simulink model "sampleModel1630_1_sub"  (R2023a)
settings: Solver=VariableStepAuto  StartTime=0.0  StopTime=10.0  RelTol=1e-3
libraries: hdlsllib x3
settings Model: Creator=user1  LastModifiedBy=user1

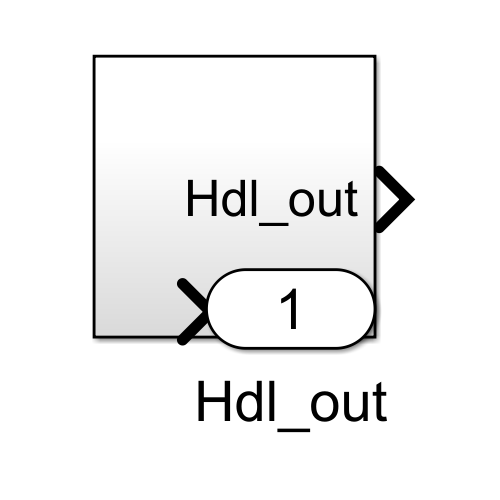
[thumbnail: Simulink's stored preview of the top-level diagram]
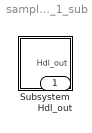
== system sampleModel1630_1_sub ==
  Subsystem : Subsystem
  Hdl_out : Outport  OutDataTypeStr=uint8

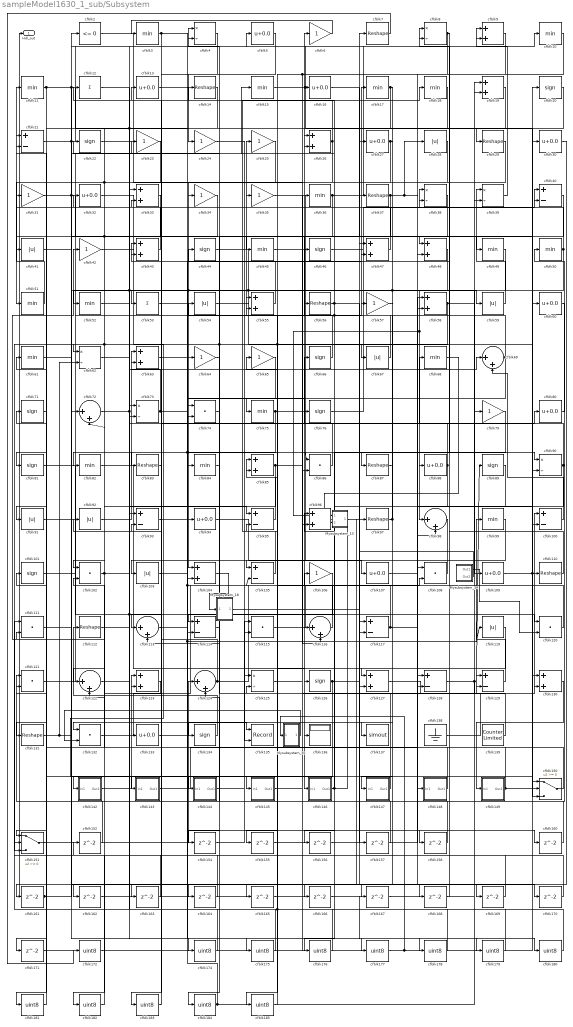
== system sampleModel1630_1_sub/Subsystem ==
  Mysubsystem_13 : Subsystem  TreatAsAtomicUnit=on  RTWFcnName=Mysubsystem_13
      settings: RTWFcnNameOpts=User specified  RTWFileNameOpts=Use function name
  Mysubsystem_18 : Subsystem  TreatAsAtomicUnit=on  RTWFcnName=Mysubsystem_18
      settings: RTWFcnNameOpts=User specified  RTWFileNameOpts=Use function name
  Mysubsystem_34 : Subsystem  TreatAsAtomicUnit=on  RTWFcnName=Mysubsystem_34
      settings: RTWFcnNameOpts=User specified  RTWFileNameOpts=Use function name
  Mysubsystem_35 : Subsystem  TreatAsAtomicUnit=on  RTWFcnName=Mysubsystem_35
      settings: RTWFcnNameOpts=User specified  RTWFileNameOpts=Use function name
  cfblk{3,10..11,15,17..18,36,45,49..52,61,68,75,82,84,99} (18 alike) : MinMax  OutDataTypeStr=uint8
  cfblk{21,40,93,95,100,105,114,117,128..129} (10 alike) : Sum  Inputs=+-  OutDataTypeStr=uint8
  cfblk{20,22,44,46,66,71,76,81,89,101,126,134} (12 alike) : Signum
  cfblk{74,86,102,108,111,115,120..121,132} (9 alike) : DotProduct  OutDataTypeStr=uint8
  cfblk{28,41,54,59,67,91..92,103,119} (9 alike) : Abs  OutDataTypeStr=uint8  SaturateOnIntegerOverflow=off
  cfblk{9,19,26,33,43,47..48,55,58,63,85,96,104,123,127,130} (16 alike) : Sum  OutDataTypeStr=uint8
  cfblk{6,23..25,31,34..35,42,57,64..65,79,106} (13 alike) : Gain  OutDataTypeStr=uint8
  cfblk{5,13,16,27,30,32,60,80,88,94,107,109,133} (13 alike) : Bias  Bias=0.0  SaturateOnIntegerOverflow=off
  cfblk{7,14,29,37,56,83,87,97,110,112,131} (11 alike) : Reshape
  cfblk{69,72,98,113,116,122,124} (7 alike) : Sum  Inputs=|++  OutDataTypeStr=uint8
  cfblk12 : Sum  Inputs=+  OutDataTypeStr=uint8
  cfblk{4,8,38..39,62,73,90,125} (8 alike) : Product  Inputs=*/  OutDataTypeStr=uint8  RndMeth=Zero  SaturateOnIntegerOverflow=on
  cfblk135 : Record  FileSettingsInternal="{\"entries\":[{\"content\":{\"excelSettings\":{\"content\":{},\"type\":\"Streamout.ExcelSettings\"}},\"type\":\"Streamout.FileSettingStorage\",\"uuid\":\"\"}],\"packageUris\":[\"http:\\/\\/schema.mathworks.com\\/mf0\\/streamout_blocks\\/R2020a\"],\"version\":\"1.0\"}"  Layout=[1 1]  SignalsInternal="{\"entries\":[{\"content\":{\"signals\":[{\"content\":{\"blockPath\":[],\"dimensions\":[1],\"domain\":\"\",\"lineColor\":\"#a2142f\",\"plots\":[1],\"port\":1,\"signalID\":29905,\"signalName\":\"cfblk73\"},\"type\":\"RecordBlkView.Signal\",\"uuid\":\"\"},{\"content\":{\"blockPath\":[],\"dimensions\":[1],\"domain\":\"\",\"lineColor\":\"#139fff\",\"plots\":[1],\"port\":2,\"signalID\":29908,\"signalName\":\"cfblk36\"},\"type\":\"RecordBlkView.Signal\",\"uuid\":\"\"}]},\"type\":\"RecordBlkView.InputSignals\",\"uuid\":\"\"}],\"packageUris\":[\"http:\\/\\/schema.mathworks.com\\/mf0\\/streamout_blocks\\/R2020a\"],\"version\":\"1.0\"}"  VisualizationBindings="{\"xyplotplugin\":{\"info\":[{\"series\":[{\"bindingParametersList\":[{\"parameter\":\"X-Axis\",\"signalID\":29905,\"signalName\":\"cfblk73\"},{\"parameter\":\"Y-Axis\",\"signalID\":29908,\"signalName\":\"cfblk36\"}],\"seriesID\":2341}],\"subplotID\":1}]}}"  CompatibilityTag=XY  st=-1
  cfblk136 : Display
  cfblk137 : ToWorkspace  VariableName=simout  SaveFormat=Timeseries  SampleTime=-1
  cfblk138 : Ground
  cfblk139 : hdlsllib/Sources/Counter Limited  uplimit=7  tsamp=-1
  cfblk142 : Subsystem
      settings: LibrarySourceBlock=|
      | hdlsllib/Ports &
      | Subsystems/Subsystem
  cfblk143 : Subsystem
      settings: LibrarySourceBlock=|
      | hdlsllib/Ports &
      | Subsystems/Subsystem
  cfblk144 : Subsystem
      settings: LibrarySourceBlock=|
      | hdlsllib/Ports &
      | Subsystems/Subsystem
  cfblk145 : Subsystem
      settings: LibrarySourceBlock=|
      | hdlsllib/Ports &
      | Subsystems/Subsystem
  cfblk146 : Subsystem
      settings: LibrarySourceBlock=|
      | hdlsllib/Ports &
      | Subsystems/Subsystem
  cfblk147 : Subsystem
      settings: LibrarySourceBlock=|
      | hdlsllib/Ports &
      | Subsystems/Subsystem
  cfblk148 : Subsystem
      settings: LibrarySourceBlock=|
      | hdlsllib/Ports &
      | Subsystems/Subsystem
  cfblk149 : Subsystem
      settings: LibrarySourceBlock=|
      | hdlsllib/Ports &
      | Subsystems/Subsystem
  cfblk150 : Switch  OutDataTypeStr=uint8  SaturateOnIntegerOverflow=off  InputSameDT=off
  cfblk151 : Switch  OutDataTypeStr=uint8  SaturateOnIntegerOverflow=off  InputSameDT=off
  cfblk{152,154..158,160..171} (18 alike) : Delay  SampleTime=1
  cfblk{172,174..185} (13 alike) : DataTypeConversion  OutDataTypeStr=uint8  SaturateOnIntegerOverflow=off  RndMeth=Floor
  cfblk2 : hdlsllib/Logic and Bit Operations/Compare To Zero  relop=<=  OutDataTypeStr=uint8
  cfblk53 : Sum  Inputs=+  OutDataTypeStr=uint8
  Hdl_out : Outport  OutDataTypeStr=uint8
  wires:
  cfblk45/1 -> cfblk107/1
  cfblk19/1 -> cfblk29/1
  cfblk5/1 -> cfblk24/1
  cfblk73/1 -> cfblk135/1, cfblk63/1
  cfblk92/1 -> cfblk63/2
  cfblk87/1 -> cfblk132/1
  cfblk37/1 -> cfblk84/1, cfblk100/2, cfblk28/1
  cfblk150/1 -> cfblk8/1
  cfblk105/1 -> cfblk18/1
  cfblk76/1 -> cfblk38/1
  cfblk101/1 -> cfblk15/1
  cfblk21/1 -> cfblk9/2, cfblk26/2, cfblk5/1
  cfblk32/1 -> cfblk145/1(In1)
  cfblk38/1 -> cfblk146/1(In1)
  cfblk93/1 -> cfblk177/1
  cfblk51/1 -> cfblk11/1
  cfblk60/1 -> cfblk121/1
  cfblk82/1 -> cfblk126/1
  cfblk138/1 -> cfblk100/1
  cfblk97/1 -> cfblk167/1, cfblk57/1
  cfblk74/1 -> cfblk14/1
  cfblk123/1 -> cfblk42/1
  cfblk43/1 -> cfblk21/1
  cfblk81/1 -> cfblk120/1
  cfblk142/1(Out1) -> cfblk123/1
  cfblk128/1 -> cfblk130/2, cfblk89/1
  cfblk15/1 -> cfblk150/2, cfblk8/2
  cfblk66/1 -> cfblk6/1
  cfblk112/1 -> cfblk33/1
  cfblk35/1 -> cfblk90/1
  cfblk36/1 -> cfblk135/2, cfblk10/1
  cfblk58/1 -> cfblk40/2, cfblk105/1, cfblk144/1(In1), cfblk151/3, cfblk72/2
  cfblk62/1 -> cfblk95/1
  cfblk2/1 -> cfblk104/1
  cfblk18/1 -> cfblk52/1
  cfblk33/1 -> cfblk51/1
  cfblk145/1(Out1) -> cfblk129/1
  cfblk12/1 -> cfblk73/1
  cfblk50/1 -> cfblk35/1, cfblk98/1, Mysubsystem_13/1(In1)
  cfblk41/1 -> cfblk59/1
  cfblk54/1 -> cfblk117/1
  cfblk59/1 -> cfblk39/1
  cfblk121/1 -> cfblk17/1
  cfblk139/1 -> cfblk22/1
  cfblk10/1 -> cfblk96/2, cfblk75/1
  cfblk89/1 -> cfblk147/1(In1)
  cfblk132/1 -> cfblk37/1
  cfblk80/1 -> cfblk50/1
  cfblk3/1 -> cfblk76/1, cfblk113/1
  cfblk122/1 -> cfblk69/1
  cfblk151/1 -> cfblk124/1
  cfblk107/1 -> cfblk128/1
  cfblk90/1 -> cfblk136/1, cfblk66/1
  cfblk28/1 -> cfblk53/1
  cfblk67/1 -> cfblk25/1
  cfblk125/1 -> cfblk36/1
  cfblk129/1 -> cfblk99/1
  cfblk131/1 -> cfblk62/2, cfblk2/1
  cfblk11/1 -> cfblk81/1, cfblk169/1, cfblk94/1, cfblk133/1
  cfblk126/1 -> cfblk181/1, cfblk108/2
  cfblk116/1 -> cfblk106/1
  cfblk124/1 -> cfblk92/1, cfblk27/1
  cfblk22/1 -> cfblk46/1
  cfblk4/1 -> cfblk83/1
  cfblk134/1 -> cfblk112/1
  cfblk34/1 -> cfblk82/1, cfblk151/1
  cfblk72/1 -> cfblk55/2, cfblk178/1, cfblk116/2
  cfblk106/1 -> cfblk114/1
  cfblk91/1 -> cfblk148/1(In1)
  cfblk69/1 -> cfblk104/2, cfblk4/2, cfblk26/1
  cfblk64/1 -> cfblk134/1
  cfblk75/1 -> cfblk102/1, cfblk90/2
  cfblk127/1 -> cfblk129/2
  cfblk42/1 -> cfblk109/1, cfblk64/1
  cfblk57/1 -> cfblk127/1
  cfblk95/1 -> cfblk85/1
  cfblk86/1 -> cfblk43/1
  cfblk65/1 -> cfblk184/1
  cfblk49/1 -> cfblk137/1, cfblk122/2, cfblk73/2
  cfblk88/1 -> cfblk116/1, cfblk68/1
  cfblk26/1 -> cfblk12/1, cfblk41/1
  cfblk120/1 -> cfblk56/1
  cfblk9/1 -> cfblk128/2
  cfblk130/1 -> cfblk149/1(In1)
  cfblk84/1 -> cfblk54/1
  cfblk20/1 -> cfblk91/1
  cfblk46/1 -> cfblk40/1
  cfblk149/1(Out1) -> cfblk102/2, cfblk30/1
  cfblk13/1 -> cfblk49/1
  cfblk44/1 -> cfblk98/2, cfblk150/1
  cfblk147/1(Out1) -> cfblk113/2
  cfblk148/1(Out1) -> cfblk31/1
  cfblk17/1 -> cfblk74/2, cfblk87/1
  cfblk55/1 -> cfblk13/1
  cfblk85/1 -> cfblk117/2, cfblk142/1(In1)
  cfblk53/1 -> cfblk150/3, cfblk86/1
  cfblk61/1 -> cfblk180/1
  cfblk31/1 -> cfblk45/1, cfblk130/1
  cfblk39/1 -> cfblk9/1
  cfblk146/1(Out1) -> cfblk166/1, cfblk96/1, cfblk97/1
  cfblk103/1 -> cfblk114/2
  cfblk108/1 -> cfblk103/1
  cfblk16/1 -> cfblk48/1
  cfblk48/1 -> cfblk122/1
  cfblk47/1 -> cfblk32/1
  cfblk27/1 -> cfblk67/1, cfblk143/1(In1)
  cfblk40/1 -> cfblk48/2
  cfblk6/1 -> cfblk3/1
  cfblk8/1 -> cfblk165/1, cfblk88/1
  cfblk143/1(Out1) -> cfblk108/1
  cfblk115/1 -> cfblk58/2
  cfblk117/1 -> cfblk170/1, cfblk55/1
  cfblk52/1 -> cfblk4/1
  cfblk102/1 -> cfblk162/1, cfblk80/1
  cfblk110/1 -> cfblk44/1
  cfblk25/1 -> cfblk131/1, cfblk62/1
  cfblk133/1 -> cfblk119/1, cfblk105/2, cfblk47/2
  cfblk109/1 -> cfblk110/1, cfblk20/1
  cfblk56/1 -> cfblk158/1, cfblk16/1
  cfblk144/1(Out1) -> cfblk125/1
  cfblk24/1 -> cfblk115/2
  cfblk29/1 -> cfblk34/1
  cfblk100/1 -> cfblk69/2
  cfblk152/1 -> cfblk121/2
  cfblk114/1 -> cfblk154/1
  cfblk154/1 -> cfblk115/1
  cfblk119/1 -> cfblk155/1
  cfblk155/1 -> cfblk58/1
  cfblk99/1 -> cfblk156/1
  cfblk156/1 -> cfblk47/1
  cfblk94/1 -> cfblk157/1
  cfblk157/1 -> cfblk95/2
  cfblk158/1 -> cfblk124/2
  cfblk113/1 -> cfblk160/1
  cfblk160/1 -> cfblk33/2
  cfblk30/1 -> cfblk161/1
  cfblk161/1 -> Hdl_out/1, cfblk72/1
  cfblk162/1 -> cfblk39/2
  cfblk14/1 -> cfblk163/1
  cfblk163/1 -> cfblk21/2
  cfblk164/1 -> cfblk123/2
  cfblk165/1 -> cfblk85/2
  cfblk167/1 -> cfblk19/1
  cfblk96/1 -> cfblk168/1
  cfblk168/1 -> cfblk38/2
  cfblk169/1 -> cfblk43/2
  cfblk170/1 -> cfblk151/2
  cfblk71/1 -> cfblk171/1
  cfblk171/1 -> cfblk86/2
  cfblk7/1 -> cfblk172/1
  cfblk172/1 -> cfblk60/1
  cfblk111/1 -> cfblk174/1
  cfblk174/1 -> cfblk101/1
  cfblk63/1 -> cfblk175/1
  cfblk175/1 -> cfblk111/1
  cfblk79/1 -> cfblk176/1
  cfblk176/1 -> cfblk111/2
  cfblk177/1 -> cfblk19/2, Mysubsystem_35/1(In1)
  cfblk178/1 -> cfblk93/1
  cfblk166/1 -> cfblk179/1
  cfblk179/1 -> cfblk93/2
  cfblk180/1 -> cfblk71/1, cfblk125/2
  cfblk181/1 -> cfblk61/1
  cfblk23/1 -> cfblk182/1
  cfblk182/1 -> cfblk152/1
  cfblk83/1 -> cfblk183/1
  cfblk183/1 -> cfblk23/1
  cfblk184/1 -> cfblk74/1, cfblk79/1
  cfblk98/1 -> cfblk185/1
  cfblk185/1 -> cfblk65/1
  cfblk68/1 -> Mysubsystem_13/2(In2)
  Mysubsystem_13/1(Out1) -> cfblk164/1
  cfblk104/1 -> Mysubsystem_18/1(In1)
  Mysubsystem_18/1(Out1) -> cfblk7/1
  Mysubsystem_34/1(Out1) -> cfblk120/2
  Mysubsystem_34/2(Out2) -> cfblk127/2
  Mysubsystem_35/1(Out1) -> cfblk132/2

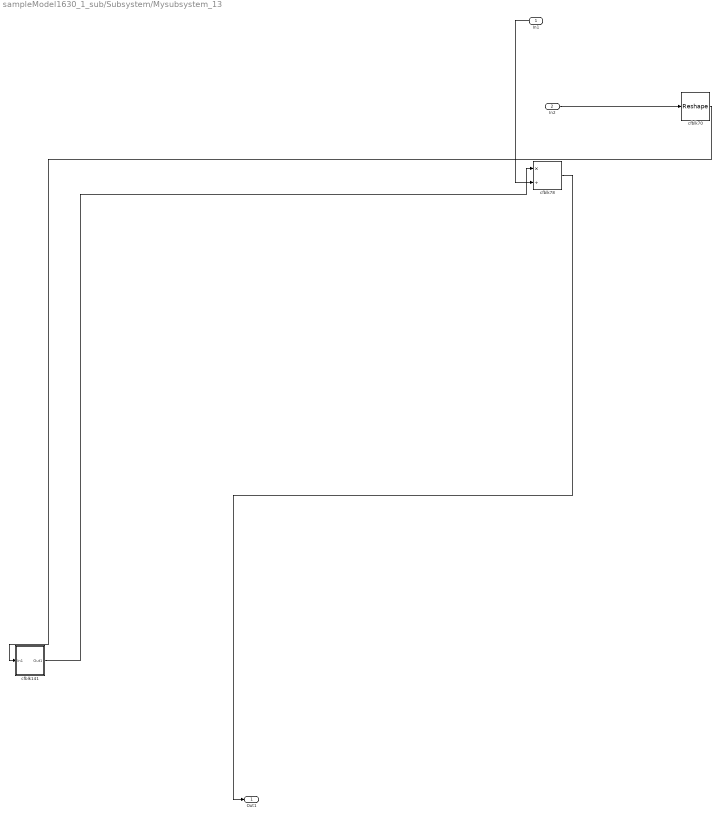
== system sampleModel1630_1_sub/Subsystem/Mysubsystem_13 ==
  In1 : Inport
  In2 : Inport  Port=2
  cfblk141 : Subsystem
      settings: LibrarySourceBlock=|
      | hdlsllib/Ports &
      | Subsystems/Subsystem
  cfblk70 : Reshape
  cfblk78 : Product  Inputs=*/  RndMeth=Zero  SaturateOnIntegerOverflow=on
  Out1 : Outport
  wires:
  In2/1 -> cfblk70/1
  cfblk78/1 -> Out1/1
  cfblk141/1(Out1) -> cfblk78/1
  cfblk70/1 -> cfblk141/1(In1)
  In1/1 -> cfblk78/2

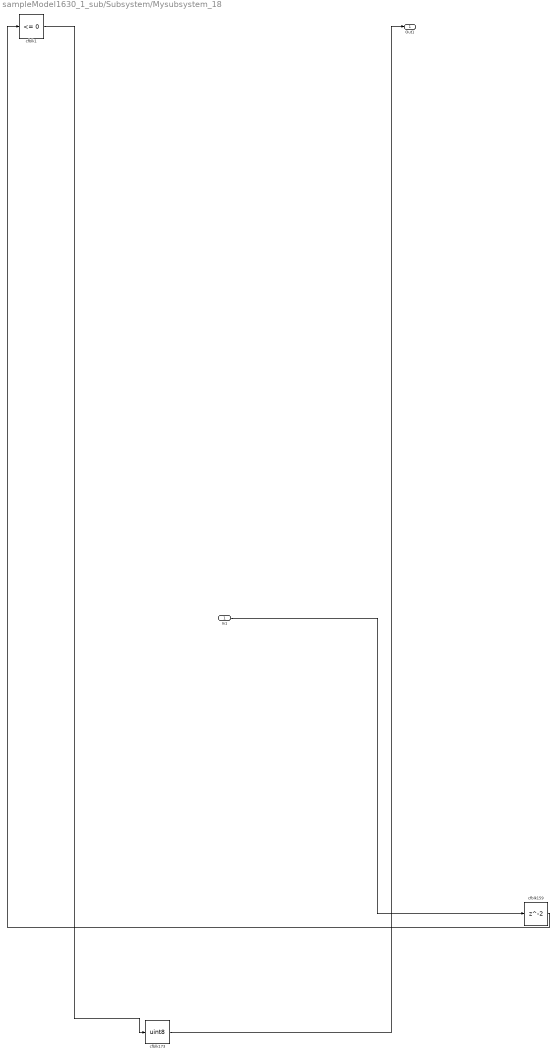
== system sampleModel1630_1_sub/Subsystem/Mysubsystem_18 ==
  In1 : Inport
  cfblk1 : hdlsllib/Logic and Bit Operations/Compare To Zero  relop=<=  OutDataTypeStr=boolean
  cfblk159 : Delay  SampleTime=1
  cfblk173 : DataTypeConversion  OutDataTypeStr=uint8  SaturateOnIntegerOverflow=off  RndMeth=Floor
  Out1 : Outport
  wires:
  In1/1 -> cfblk159/1
  cfblk173/1 -> Out1/1
  cfblk159/1 -> cfblk1/1
  cfblk1/1 -> cfblk173/1

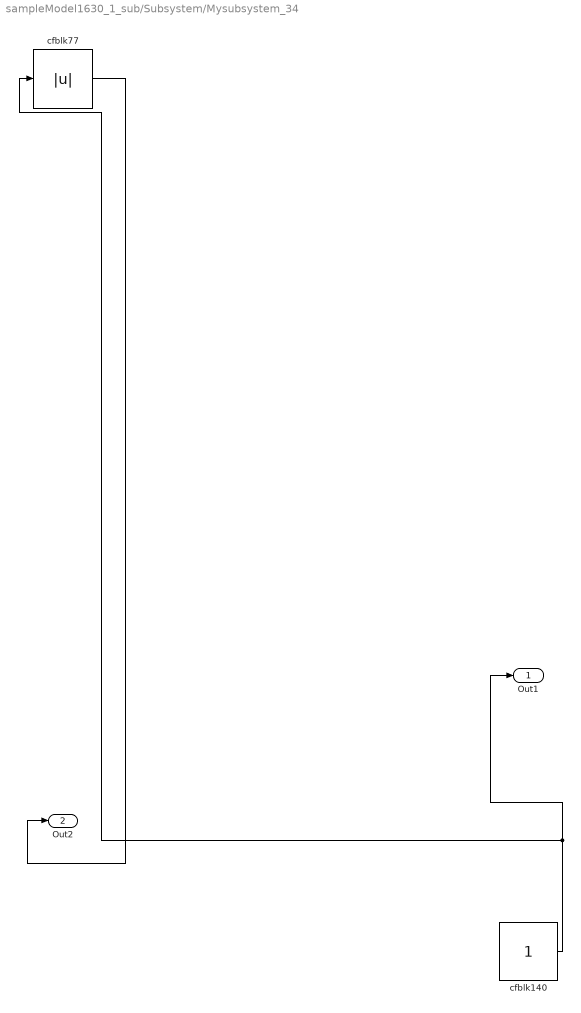
== system sampleModel1630_1_sub/Subsystem/Mysubsystem_34 ==
  cfblk140 : Constant  SampleTime=-1
  cfblk77 : Abs  SaturateOnIntegerOverflow=off
  Out1 : Outport
  Out2 : Outport  Port=2
  wires:
  cfblk77/1 -> Out2/1
  cfblk140/1 -> cfblk77/1, Out1/1

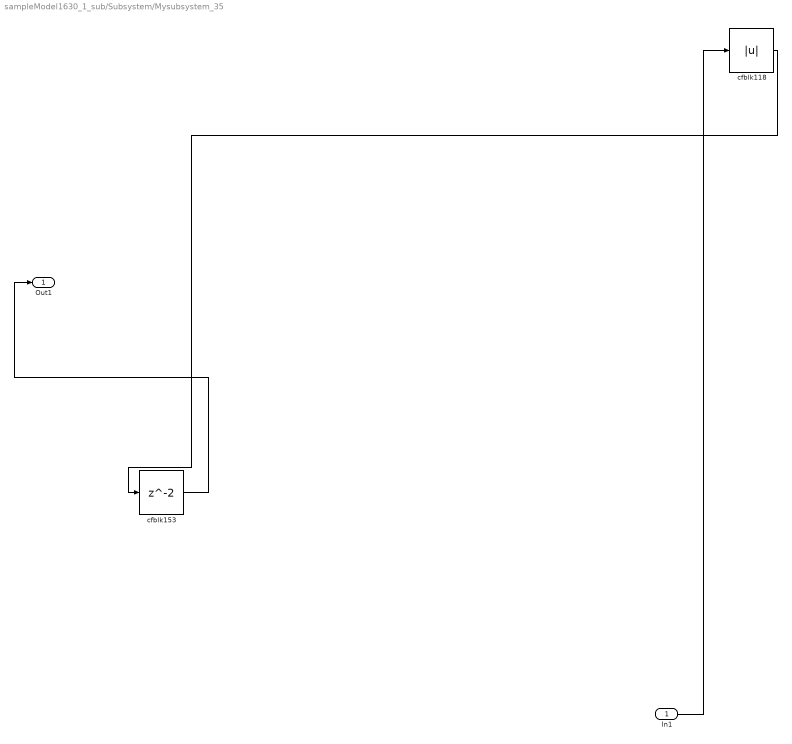
== system sampleModel1630_1_sub/Subsystem/Mysubsystem_35 ==
  In1 : Inport
  cfblk118 : Abs  SaturateOnIntegerOverflow=off
  cfblk153 : Delay  SampleTime=1
  Out1 : Outport
  wires:
  cfblk153/1 -> Out1/1
  In1/1 -> cfblk118/1
  cfblk118/1 -> cfblk153/1

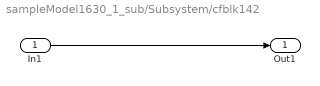
== system sampleModel1630_1_sub/Subsystem/cfblk142 ==
  In1 : Inport
  Out1 : Outport
  wires:
  In1/1 -> Out1/1

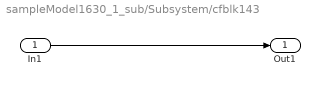
== system sampleModel1630_1_sub/Subsystem/cfblk143 ==
  In1 : Inport
  Out1 : Outport
  wires:
  In1/1 -> Out1/1

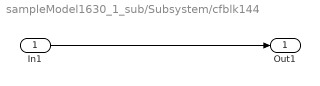
== system sampleModel1630_1_sub/Subsystem/cfblk144 ==
  In1 : Inport
  Out1 : Outport
  wires:
  In1/1 -> Out1/1

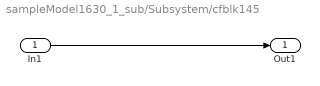
== system sampleModel1630_1_sub/Subsystem/cfblk145 ==
  In1 : Inport
  Out1 : Outport
  wires:
  In1/1 -> Out1/1

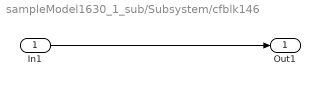
== system sampleModel1630_1_sub/Subsystem/cfblk146 ==
  In1 : Inport
  Out1 : Outport
  wires:
  In1/1 -> Out1/1

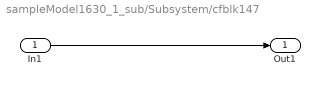
== system sampleModel1630_1_sub/Subsystem/cfblk147 ==
  In1 : Inport
  Out1 : Outport
  wires:
  In1/1 -> Out1/1

== system sampleModel1630_1_sub/Subsystem/cfblk148 ==
  In1 : Inport
  Out1 : Outport
  wires:
  In1/1 -> Out1/1

== system sampleModel1630_1_sub/Subsystem/cfblk149 ==
  In1 : Inport
  Out1 : Outport
  wires:
  In1/1 -> Out1/1

== system sampleModel1630_1_sub/Subsystem/Mysubsystem_13/cfblk141 ==
  In1 : Inport
  Out1 : Outport
  wires:
  In1/1 -> Out1/1
